simulink model "metoda1_bezposrednia"  (R2017b)
settings: Solver=VariableStepAuto  StartTime=0.0  StopTime=10  RelTol=1e-3
values from neighbouring files (symbols this model uses):
  A1 = [3.22791678547  -1.44925930399  0.17377394345; 1  0  0; 0  1  0]    [matlab.mat]
  C1 = [0.260707487539 -0.289205764977 0.0761198486843]    [matlab.mat]
  Tp = 0.25    [matlab.mat]
  x_start = [3 -2 1]    [matlab.mat]
settings Model: Creator=gulin  LastModifiedBy=gulin

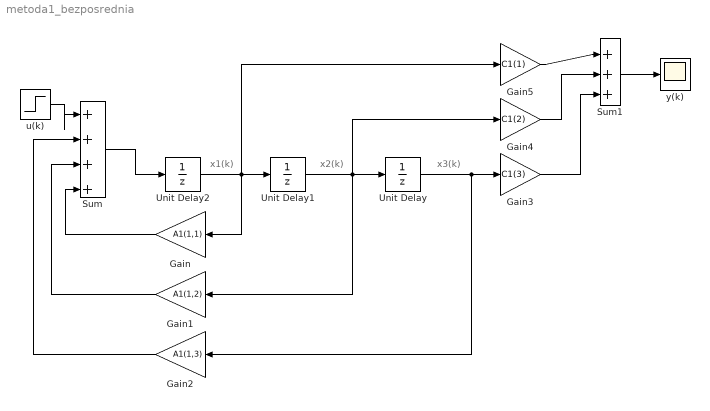
== system metoda1_bezposrednia ==
  note: x3(k)
  note: x2(k)
  note: x1(k)
  Gain : Gain  Gain=A1(1,1)
  Gain1 : Gain  Gain=A1(1,2)
  Gain2 : Gain  Gain=A1(1,3)
  Gain3 : Gain  Gain=C1(3)
  Gain4 : Gain  Gain=C1(2)
  Gain5 : Gain  Gain=C1(1)
  Sum : Sum  Inputs=|++++
  Sum1 : Sum  Inputs=|+++
  Unit Delay : UnitDelay  InitialCondition=x_start(3)  SampleTime=Tp
  Unit Delay1 : UnitDelay  InitialCondition=x_start(2)  SampleTime=Tp
  Unit Delay2 : UnitDelay  InitialCondition=x_start(1)  SampleTime=Tp
  u(k) : Step  SampleTime=0
  "y(k) " : Scope
  wires:
  Sum/1 -> Unit Delay2/1
  Unit Delay2/1 -> Gain5/1, Unit Delay1/1, Gain/1
  Gain/1 -> Sum/4
  Gain1/1 -> Sum/3
  Unit Delay1/1 -> Unit Delay/1, Gain1/1, Gain4/1
  Unit Delay/1 -> Gain3/1, Gain2/1
  Gain2/1 -> Sum/2
  Gain3/1 -> Sum1/3
  Gain4/1 -> Sum1/2
  Gain5/1 -> Sum1/1
  Sum1/1 -> "y(k) "/1
  u(k)/1 -> Sum/1
